simulink model "dev_UnitTest"  (R2020b)
settings: Solver=VariableStepAuto  StartTime=0.0  StopTime=1500  RelTol=1e-3
libraries: simulink_extras x3, simulink x1
settings Model: Creator=Mr_Li  LastModifiedBy=Mr_Li

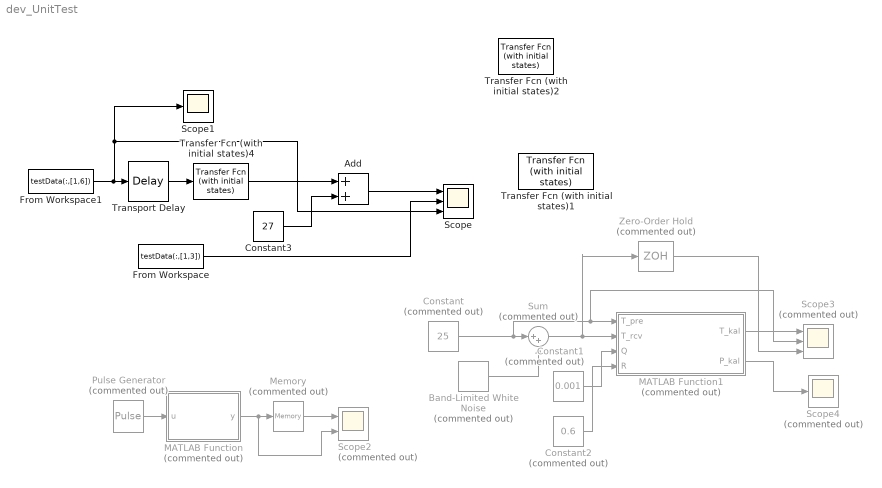
== system dev_UnitTest ==
  Add : Sum
  Band-Limited White Noise : simulink/Sources/Band-Limited White Noise  Commented=on  Cov=[1]  Ts=0.1  seed=[23341]
  Constant : Constant  Commented=on  Value=25
  Constant1 : Constant  Commented=on  Value=0.001
  Constant2 : Constant  Commented=on  Value=0.6
  Constant3 : Constant  Value=27
  From Workspace : FromWorkspace  VariableName=testData(:,[1,3])
  From Workspace1 : FromWorkspace  VariableName=testData(:,[1,6])
  MATLAB Function : MATLAB Function  Commented=on  TreatAsAtomicUnit=on
  MATLAB Function1 : MATLAB Function  Commented=on  TreatAsAtomicUnit=on
  Memory : Memory  Commented=on  InheritSampleTime=on  LinearizeMemory=on  LinearizeAsDelay=on
  Pulse Generator : DiscretePulseGenerator  Commented=on  Period=10
  Scope : Scope  NumInputPorts=3
  Scope1 : Scope
  Scope2 : Scope  Commented=on  NumInputPorts=2
  Scope3 : Scope  Commented=on  NumInputPorts=3
  Scope4 : Scope  Commented=on
  Sum : Sum  Commented=on  Inputs=|++
  Transfer Fcn (with initial states)1 : simulink_extras/Additional Linear/Transfer Fcn (with initial states)  N=[2]  D=[4 31.6 1]  X0=0
  Transfer Fcn (with initial states)2 : simulink_extras/Additional Linear/Transfer Fcn (with initial states)  N=[6.5]  D=[110 1]  X0=0
  Transfer Fcn (with initial states)4 : simulink_extras/Additional Linear/Transfer Fcn (with initial states)  N=[3.6]  D=[40 1]  X0=0
  Transport Delay : TransportDelay  DelayTime=5
  Zero-Order Hold : ZeroOrderHold  Commented=on
  wires:
  From Workspace1/1 -> Scope/3, Scope1/1, Transport Delay/1
  From Workspace/1 -> Scope/2
  Transport Delay/1 -> Transfer Fcn (with initial states)4/1
  Pulse Generator/1 -> MATLAB Function/1(u)
  Memory/1 -> Scope2/1
  MATLAB Function/1(y) -> Scope2/2, Memory/1
  Sum/1 -> Zero-Order Hold/1, MATLAB Function1/2(T_rcv)
  Constant/1 -> Scope3/2, MATLAB Function1/1(T_pre), Sum/1
  Band-Limited White Noise/1 -> Sum/2
  Constant1/1 -> MATLAB Function1/3(Q)
  Constant2/1 -> MATLAB Function1/4(R)
  MATLAB Function1/1(T_kal) -> Scope3/1
  Zero-Order Hold/1 -> Scope3/3
  MATLAB Function1/2(P_kal) -> Scope4/1
  Constant3/1 -> Add/2
  Transfer Fcn (with initial states)4/1 -> Add/1
  Add/1 -> Scope/1

== matlab function dev_UnitTest/MATLAB Function1 ==
  settings: updateMethod=DISCRETE  sampleTime=1
  data: T_pre input; T_kal output; T_rcv input; P_kal output; Q input; R input
function [T_kal,P_kal] = fcn(T_pre,T_rcv,Q,R)
persistent P_previous;
if(isempty(P_previous))
    P_previous=1;
end
    P_pre=P_previous+Q;
    K=P_pre/(P_pre+R);%K(k)???????
    T_kal=T_pre+K*(T_rcv-T_pre);
    P_kal=P_pre-(K*P_pre);
    P_previous=P_kal;
end

== matlab function dev_UnitTest/MATLAB Function ==
  settings: updateMethod=DISCRETE  sampleTime=1
  data: u input; y output
function y = fcn(u)

persistent u0;

if(isempty(u0))
    u0=2;
else
    u0=u;
end

y = u0;
